simulink model "VCU_Control"  (R2026a)
settings: Solver=VariableStepAuto
undefined symbols (not defined in the file): VCU_batt_ocv_table, VCU_batt_parallel_cells, VCU_batt_r0_table, VCU_batt_series_cells, VCU_batt_soc_bp_ocv, VCU_batt_soc_bp_r0, VCU_batt_temp_bp_r0, VCU_cell_voltage_min, VCU_derate_Vfull, VCU_derate_Vmin, VCU_drivetrain_efficiency, VCU_max_power, VCU_omega_floor, VCU_torque_fall_rate, VCU_torque_lpf_tau, VCU_torque_rise_rate
libraries: eeGeneralControl x1
settings Model: Creator=renil  LastModifiedBy=renil

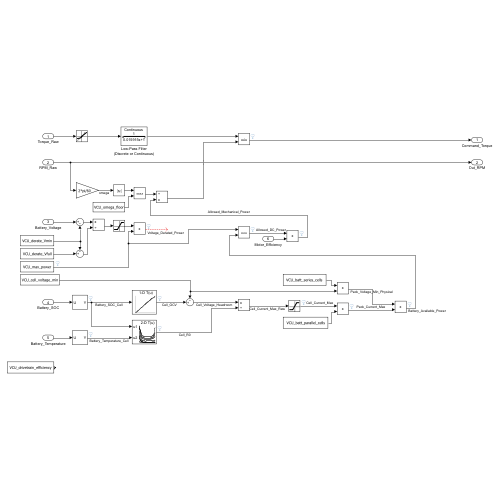
[thumbnail: Simulink's stored preview of the top-level diagram]
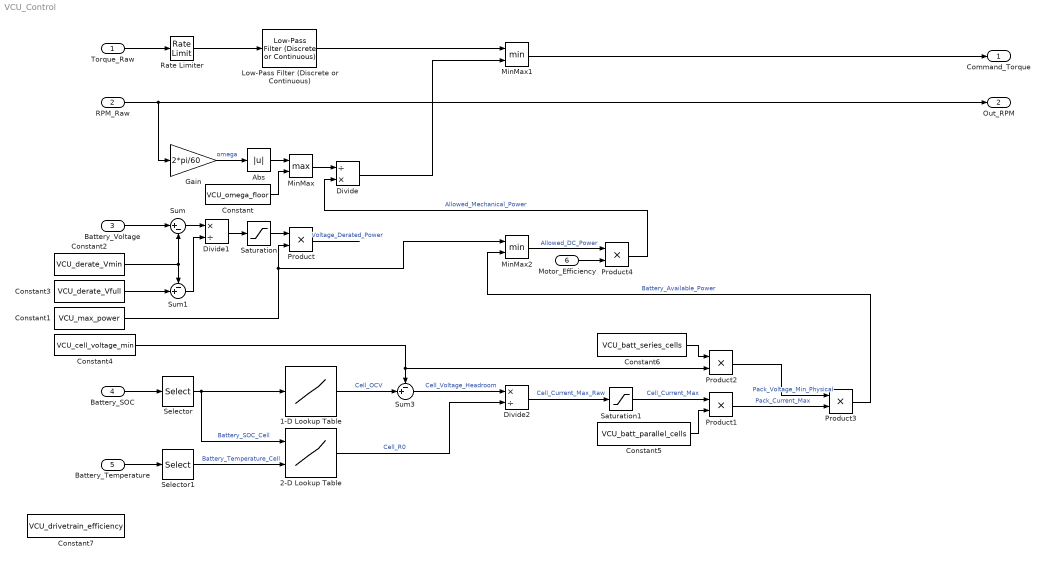
== system VCU_Control ==
  Torque_Raw : Inport
  RPM_Raw : Inport  Port=2
  Battery_Voltage : Inport  Port=3
  Battery_SOC : Inport  Port=4
  Battery_Temperature : Inport  Port=5
  Motor_Efficiency : Inport  Port=6
  1-D Lookup Table : Lookup_n-D  NumberOfTableDimensions=1  BreakpointsForDimension1=VCU_batt_soc_bp_ocv  Table=VCU_batt_ocv_table  InternalRulePriority=Speed  RndMeth=Simplest
  2-D Lookup Table : Lookup_n-D  BreakpointsForDimension1=VCU_batt_soc_bp_r0  BreakpointsForDimension2=VCU_batt_temp_bp_r0  Table=VCU_batt_r0_table  InternalRulePriority=Speed  RndMeth=Simplest
      settings: InputPortMap=u0,u1
  Abs : Abs  SaturateOnIntegerOverflow=off
  Constant : Constant  Value=VCU_omega_floor
  Constant1 : Constant  Value=VCU_max_power
  Constant2 : Constant  Value=VCU_derate_Vmin
  Constant3 : Constant  Value=VCU_derate_Vfull
  Constant4 : Constant  Value=VCU_cell_voltage_min
  Constant5 : Constant  Value=VCU_batt_parallel_cells
  Constant6 : Constant  Value=VCU_batt_series_cells
  Constant7 : Constant  Value=VCU_drivetrain_efficiency
  Divide : Product  Inputs=/*
  Divide1 : Product  Inputs=*/
  Divide2 : Product  Inputs=*/
  Gain : Gain  Gain=2*pi/60
  Low-Pass Filter (Discrete or Continuous) : eeGeneralControl/Low-Pass Filter (Discrete or Continuous)  K=1  T=VCU_torque_lpf_tau  B=inf  A=-inf  init_option=Inherited from block input  x0=0  Ts=0
  MinMax : MinMax  Function=max  Inputs=2
  MinMax1 : MinMax  Inputs=2
  MinMax2 : MinMax  Inputs=2
  Product{,1..4} (5 alike) : Product
  Rate Limiter : RateLimiter  RisingSlewLimit=VCU_torque_rise_rate  FallingSlewLimit=VCU_torque_fall_rate  SampleTimeMode=inherited
  Saturation : Saturate  UpperLimit=1  LowerLimit=0
  Saturation1 : Saturate  UpperLimit=inf  LowerLimit=0
  Selector : Selector  InputPortWidth=10  IndexOptions=Index vector (dialog)  Indices=1  OutputSizes=1
  Selector1 : Selector  InputPortWidth=10  IndexOptions=Index vector (dialog)  Indices=1  OutputSizes=1
  Sum : Sum  Inputs=|+-
  Sum1 : Sum  Inputs=-+|
  Sum3 : Sum  Inputs=-+|
  Command_Torque : Outport
  Out_RPM : Outport  Port=2
  wires:
  RPM_Raw/1 -> Out_RPM/1, Gain/1
  Torque_Raw/1 -> Rate Limiter/1
  Rate Limiter/1 -> Low-Pass Filter (Discrete or Continuous)/1
  Gain/1 -> Abs/1  "omega"
  Abs/1 -> MinMax/1
  Constant/1 -> MinMax/2
  MinMax/1 -> Divide/1
  MinMax1/1 -> Command_Torque/1
  Divide/1 -> MinMax1/2
  Low-Pass Filter (Discrete or Continuous)/1 -> MinMax1/1
  Battery_Voltage/1 -> Sum/1
  Constant2/1 -> Sum1/1, Sum/2
  Sum/1 -> Divide1/1
  Divide1/1 -> Saturation/1
  Product/1 -> ?  "Voltage_Derated_Power"
  Constant3/1 -> Sum1/2
  Sum1/1 -> Divide1/2
  Saturation/1 -> Product/1
  Constant1/1 -> Product/2, MinMax2/1
  Battery_SOC/1 -> Selector/1
  Selector/1 -> 2-D Lookup Table/1, 1-D Lookup Table/1  "Battery_SOC_Cell"
  Battery_Temperature/1 -> Selector1/1
  Selector1/1 -> 2-D Lookup Table/2  "Battery_Temperature_Cell"
  1-D Lookup Table/1 -> Sum3/2  "Cell_OCV"
  2-D Lookup Table/1 -> Divide2/2  "Cell_R0"
  Constant4/1 -> Sum3/1, Product2/2
  Sum3/1 -> Divide2/1  "Cell_Voltage_Headroom"
  Divide2/1 -> Saturation1/1  "Cell_Current_Max_Raw"
  Saturation1/1 -> Product1/1  "Cell_Current_Max"
  Constant5/1 -> Product1/2
  Product1/1 -> Product3/2  "Pack_Current_Max"
  Product2/1 -> Product3/1  "Pack_Voltage_Min_Physical"
  Product3/1 -> MinMax2/2  "Battery_Available_Power"
  Constant6/1 -> Product2/1
  MinMax2/1 -> Product4/1  "Allowed_DC_Power"
  Product4/1 -> Divide/2  "Allowed_Mechanical_Power"
  Motor_Efficiency/1 -> Product4/2
